simulink subsystem "RoboRio_Controls_sub"  (R2023b)
settings: Solver=VariableStepAuto  StartTime=0.0  StopTime=10.0  RelTol=1e-3
undefined symbols (not defined in the file): All_Num_Poses, All_Paths, Autonomous, Autonomous_lib, Climber_DutyCycle_Neg, Climber_DutyCycle_Pos, FloorDistance, Odometry_IC_X, Odometry_IC_Y
libraries: simulink x5, Disabled_lib x1, Teleop_lib x1, Test_lib x1
(part 1 of 2)
settings Model: Creator=USER  LastModifiedBy=FIRSTMentor

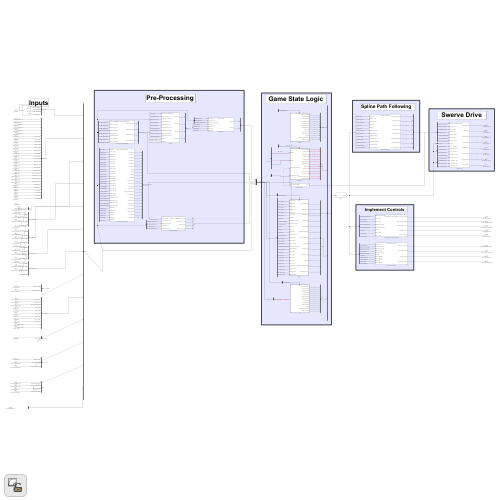
[thumbnail: Simulink's stored preview of the top-level diagram]
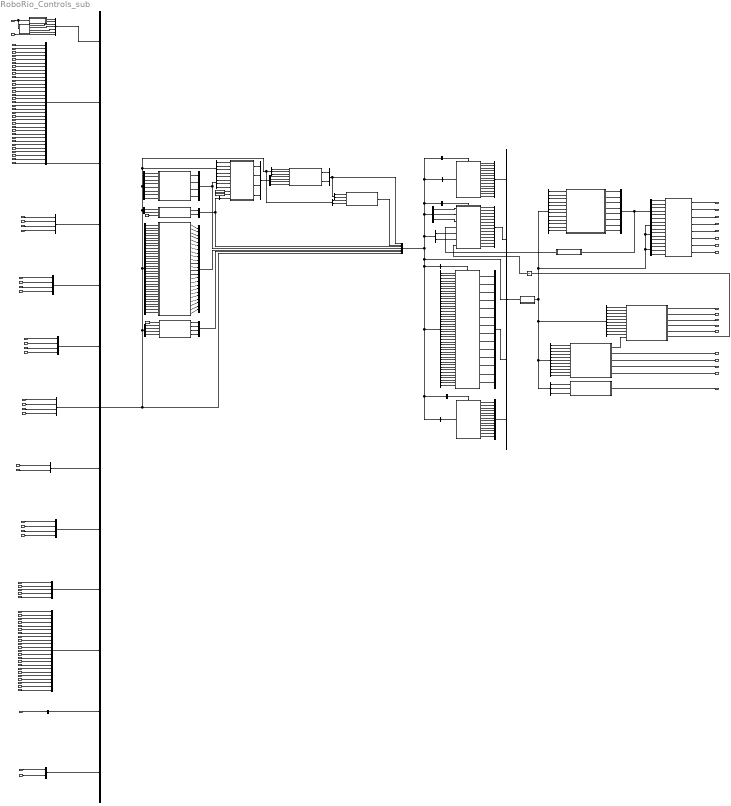
== system RoboRio_Controls_sub ==
  note: Game State Logic
  note: Swerve Drive
  note: Inputs
  note: Pre-Processing
  note: Spline Path
      | Following
  note: Implement Controls
  GameState : Inport
  IsRedAlliance : Inport  Port=2
  Joystick_Left_X : Inport  Port=3
  Joystick_Left_Y : Inport  Port=4
  Joystick_Left_Z : Inport  Port=5
  Joystick_Right_X : Inport  Port=6
  Joystick_Right_Y : Inport  Port=7
  Joystick_Right_Z : Inport  Port=8
  Joystick_Left_B1 : Inport  Port=9
  Joystick_Left_B2 : Inport  Port=10
  Joystick_Left_B3 : Inport  Port=11
  Joystick_Left_B4 : Inport  Port=12
  Joystick_Left_B7 : Inport  Port=13
  Joystick_Left_B8 : Inport  Port=14
  Joystick_Left_B10 : Inport  Port=15
  Joystick_Left_POV : Inport  Port=16
  Joystick_Right_B1 : Inport  Port=17
  Joystick_Right_B2 : Inport  Port=18
  Joystick_Right_B3 : Inport  Port=19
  Joystick_Right_B4 : Inport  Port=20
  Joystick_Right_POV : Inport  Port=21
  Joystick_Right_B7 : Inport  Port=22
  Joystick_Right_B8 : Inport  Port=23
  Joystick_Right_B10 : Inport  Port=24
  Joystick_Right_B14 : Inport  Port=25
  Gamepad_Stick_Left_X : Inport  Port=26
  Gamepad_Stick_Left_Y : Inport  Port=27
  Gamepad_Stick_Right_X : Inport  Port=28
  Gamepad_Stick_Right_Y : Inport  Port=29
  Gamepad_B1_A : Inport  Port=30
  Gamepad_B4_Y : Inport  Port=31
  Gamepad_LB : Inport  Port=32
  Gamepad_LT : Inport  Port=33
  Gamepad_RB : Inport  Port=34
  Gamepad_RT : Inport  Port=35
  Gyro_Angle : Inport  Port=36
  FL_Drive_Motor_Speed : Inport  Port=37
  FR_Drive_Motor_Speed : Inport  Port=38
  BL_Drive_Motor_Speed : Inport  Port=39
  BR_Drive_Motor_Speed : Inport  Port=40
  FL_Drive_Motor_Rev : Inport  Port=41
  FR_Drive_Motor_Rev : Inport  Port=42
  BL_Drive_Motor_Rev : Inport  Port=43
  BR_Drive_Motor_Rev : Inport  Port=44
  FL_Steer_Module_Rev : Inport  Port=45
  FR_Steer_Module_Rev : Inport  Port=46
  BL_Steer_Module_Rev : Inport  Port=47
  BR_Steer_Module_Rev : Inport  Port=48
  FL_Steer_Module_Offset : Inport  Port=49
  FR_Steer_Module_Offset : Inport  Port=50
  BL_Steer_Module_Offset : Inport  Port=51
  BR_Steer_Module_Offset : Inport  Port=52
  Is_Absolute_Steering : Inport  Port=53
  Is_Absolute_Translation : Inport  Port=54
  Intake_TOF_Dist : Inport  Port=55
  Shooter_TOF_Dist : Inport  Port=56
  Shooter_Left_Motor_RPM : Inport  Port=57
  Shooter_Right_Motor_RPM : Inport  Port=58
  Encoder_Revs_Back_Lower : Inport  Port=59
  Encoder_Revs_Back_Upper : Inport  Port=60
  Encoder_Revs_Front : Inport  Port=61
  Encoder_Revs_Ball_Screw : Inport  Port=62
  Encoder_Revs_Climber : Inport  Port=63
  Photon_Est_Pose_X : Inport  Port=64
  Photon_Est_Pose_Y : Inport  Port=65
  Photon_Est_Pose_Ambiguity : Inport  Port=66
  AT_Tag_4_Yaw : Inport  Port=67
  AT_Tag_5_Yaw : Inport  Port=68
  AT_Tag_6_Yaw : Inport  Port=69
  AT_Tag_7_Yaw : Inport  Port=70
  AT_Tag_11_Yaw : Inport  Port=71
  AT_Tag_12_Yaw : Inport  Port=72
  AT_Tag_13_Yaw : Inport  Port=73
  AT_Tag_14_Yaw : Inport  Port=74
  AT_Tag_15_Yaw : Inport  Port=75
  AT_Tag_16_Yaw : Inport  Port=76
  AT_Tag_4_Found : Inport  Port=77
  AT_Tag_5_Found : Inport  Port=78
  AT_Tag_6_Found : Inport  Port=79
  AT_Tag_7_Found : Inport  Port=80
  Line_Sensor_TOF_Range : Inport  Port=81
  AT_Tag_11_Found : Inport  Port=82
  AT_Tag_12_Found : Inport  Port=83
  AT_Tag_13_Found : Inport  Port=84
  AT_Tag_14_Found : Inport  Port=85
  AT_Tag_15_Found : Inport  Port=86
  AT_Tag_16_Found : Inport  Port=87
  Priority_List : Inport  Port=88
  Auto_ID : Inport  Port=89
  Arm_Length_Calculation : Subsystem  ReferencedSubsystem=Arm_Length_Calculation
  Autonomous : Subsystem  AncestorBlock=Autonomous_lib/Autonomous  TreatAsAtomicUnit=on
  Bus Creator : BusCreator  Inputs=7
  Bus Creator{1..2,4,12} (4 alike) : BusCreator  Inputs=14
  Bus Creator{10,19..20,26} (4 alike) : BusCreator  Inputs=2
  Bus Creator11 : BusCreator  Inputs=13
  Bus Creator13 : BusCreator  Inputs=8
  Bus Creator{7..9,14..16,21,23} (8 alike) : BusCreator  Inputs=4
  Bus Creator17 : BusCreator  Inputs=7
  Bus Creator18 : BusCreator  Inputs=23
  Bus Creator22 : BusCreator  Inputs=5
  Bus Creator24 : BusCreator  Inputs=24
  Bus Creator25 : BusCreator  Inputs=1
  Bus Creator3 : BusCreator  Inputs=5
  Bus Creator5 : BusCreator  Inputs=33
  Bus Creator6 : BusCreator  Inputs=1
  Bus Selector : BusSelector  OutputSignals=Steering_Abs_Cmd_SPF,Steering_Rel_Cmd_SPF,Translation_Speed_SPF,Translation_Angle_SPF,Is_Absolute_Translation_SPF,Is_Absolute_Steering_SPF,Gyro_Angle_Adjustment_SPF
  Bus Selector1 : BusSelector  OutputSignals=Odom_Position_X,Odom_Position_Y,Odom_Delta_X,Odom_Delta_Y
  Bus Selector10 : BusSelector  OutputSignals=PreProcessing.Gyro.Gyro_Angle
  Bus Selector11 : BusSelector  OutputSignals=State_Request_Arm,PreProcessing.Arms.Back_Lower_Arm_Length,PreProcessing.Arms.Back_Upper_Arm_Length,PreProcessing.Arms.Front_Arm_Length,PreProcessing.Arms.Ball_Screw_Arm_Length,PreProcessing.Distance_Speaker,Test_Mode,PreProcessing.Human_Inputs.Test_DC_BackUpper,PreProcessing.Human_Inputs.Test_DC_BackLower,PreProcessing.Human_Inputs.Test_DC_Front,PreProcessing.Human_Inputs.Test_DC_BallScrew
  Bus Selector12 : BusSelector  OutputSignals=Human_Inputs.Climber_Cmd_Direction
  Bus Selector13 : BusSelector  OutputSignals=Game_States.GameState,Game_States.Prev_GameState,Human_Inputs.Joystick_Left_X,Human_Inputs.Joystick_Left_Y,Human_Inputs.Joystick_Left_Z,Human_Inputs.Joystick_Right_X,Human_Inputs.Joystick_Right_Y,Human_Inputs.Joystick_Right_Z,Human_Inputs.Joystick_Left_B1,Human_Inputs.Joystick_Left_B2,Human_Inputs.Joystick_Left_B3,Human_Inputs.Joystick_Left_B4,Human_Inputs.Joystick_Left_B7,Human_Inputs.Joystick_Left_B8,Human_Inputs.Joystick_Left_B10,Human_Inputs.Joystick_Left_POV,Human_Inputs.Joystick_Right_B1,Human_Inputs.Joystick_Right_B2,Human_Inputs.Joystick_Right_B3,Human_Inputs.Joystick_Right_B4,Human_Inputs.Joystick_Right_POV,Human_Inputs.Joystick_Right_B7,Human_Inputs.Joystick_Right_B8,Human_Inputs.Joystick_Right_B10,Human_Inputs.Joystick_Right_B14,Human_Inputs.Gamepad_Stick_Left_X,Human_Inputs.Gamepad_Stick_Left_Y,Human_Inputs.Gamepad_Stick_Right_X,Human_Inputs.Gamepad_Stick_Right_Y,Human_Inputs.Gamepad_B1_A,Human_Inputs.Gamepad_B4_Y,Human_Inputs.Gamepad_LB,Human_Inputs.Gamepad_LT,Human_Inputs.Gamepad_RB,Human_Inputs.Gamepad_RT
  Bus Selector14 : BusSelector  OutputSignals=Human_Inputs.State_Request_Arm
  Bus Selector15 : BusSelector  OutputSignals=PreProcessing.Inputs.Game_States.GameState,Climber_Cmd_Direction,PreProcessing.Inputs.Arms.Encoder_Revs_Climber
  Bus Selector16 : BusSelector  OutputSignals=Photon_Estimates.AT_Tag_4_Found,Photon_Estimates.AT_Tag_7_Found
  Bus Selector17 : BusSelector  OutputSignals=IMU_Sensor.Gyro_Angle_deg,Game_States.IsRedAlliance
  Bus Selector18 : BusSelector  OutputSignals=Inputs.Autonomus_Input.Auto_ID,Inputs.Autonomus_Input.Priority_List
  Bus Selector19 : BusSelector  OutputSignals=Gyro_Angle_Field
  Bus Selector2 : BusSelector  OutputSignals=Inputs.Game_States.Game_State_Teleop
  Bus Selector20 : BusSelector  OutputSignals=KF_Position_X,KF_Position_Y
  Bus Selector3 : BusSelector  OutputSignals=Photon_Estimates.Photon_Est_Pose_X,Photon_Estimates.Photon_Est_Pose_Y,Photon_Estimates.Photon_Est_Pose_Ambiguity
  Bus Selector4 : BusSelector  OutputSignals=Inputs.Game_States.Game_State_Auto
  Bus Selector40 : BusSelector  OutputSignals=Drive_Motor_Revs.FL_Drive_Motor_Rev,Drive_Motor_Revs.FR_Drive_Motor_Rev,Drive_Motor_Revs.BL_Drive_Motor_Rev,Drive_Motor_Revs.BR_Drive_Motor_Rev
  Bus Selector41 : BusSelector  OutputSignals=Human_Inputs.Drive_Joystick_X,Human_Inputs.Drive_Joystick_Y,Human_Inputs.Drive_Joystick_Z,Human_Inputs.Drive_Joystick_Z_Mode,Human_Inputs.Steer_Joystick_X,Human_Inputs.Steer_Joystick_Y,Human_Inputs.Steer_Joystick_Z,Human_Inputs.Is_Boosting,Inputs.Motion_Control_Modes.Is_Absolute_Translation,Inputs.Motion_Control_Modes.Is_Absolute_Steering,Human_Inputs.Align_Trap,Human_Inputs.Align_Amp,Human_Inputs.Align_Speaker,Human_Inputs.Face_Toward_Driver,Human_Inputs.Face_Right_Driver,Human_Inputs.Face_Left_Driver,Human_Inputs.Face_Away_Driver,Human_Inputs.State_Request_Intake_Shooter,Human_Inputs.State_Request_Arm,Human_Inputs.Climber_Cmd_Direction,Inputs.Photon_Estimates.AT_Tag_4_Yaw,Inputs.Photon_Estimates.AT_Tag_5_Yaw,Inputs.Photon_Estimates.AT_Tag_6_Yaw,Inputs.Photon_Estimates.AT_Tag_7_Yaw,Inputs.Photon_Estimates.AT_Tag_11_Yaw,Inputs.Photon_Estimates.AT_Tag_12_Yaw,Inputs.Photon_Estimates.AT_Tag_13_Yaw,Inputs.Photon_Estimates.AT_Tag_14_Yaw,Inputs.Photon_Estimates.AT_Tag_15_Yaw,Inputs.Photon_Estimates.AT_Tag_16_Yaw,Inputs.Photon_Estimates.AT_Tag_4_Found,Inputs.Photon_Estimates.AT_Tag_5_Found,Inputs.Photon_Estimates.AT_Tag_6_Found,Inputs.Photon_Estimates.AT_Tag_7_Found,Inputs.Photon_Estimates.AT_Tag_11_Found,Inputs.Photon_Estimates.AT_Tag_12_Found,Inputs.Photon_Estimates.AT_Tag_13_Found,Inputs.Photon_Estimates.AT_Tag_14_Found,Inputs.Photon_Estimates.AT_Tag_15_Found,Inputs.Photon_Estimates.AT_Tag_16_Found,EKF.KF_Position_X,EKF.KF_Position_Y,Inputs.Photon_Estimates.Photon_Est_Pose_Ambiguity,Distance_Speaker,Inputs.Game_States.IsRedAlliance
  Bus Selector5 : BusSelector  OutputSignals=State_Request_Intake_Shooter,PreProcessing.Inputs.Intake_and_Shooter.Intake_TOF_Dist,PreProcessing.Inputs.Intake_and_Shooter.Shooter_TOF_Dist,PreProcessing.Inputs.Intake_and_Shooter.Shooter_Left_Motor_RPM,PreProcessing.Inputs.Intake_and_Shooter.Shooter_Right_Motor_RPM,Test_Mode,PreProcessing.Human_Inputs.Test_DC_Intake,PreProcessing.Human_Inputs.Test_DC_Shooter,PreProcessing.Distance_Speaker,PreProcessing.Arms.Front_Arm_Length
  Bus Selector50 : BusSelector  OutputSignals=PreProcessing.Inputs.Drive_Motor_Speeds.FL_Drive_Motor_Speed,PreProcessing.Inputs.Drive_Motor_Speeds.FR_Drive_Motor_Speed,PreProcessing.Inputs.Drive_Motor_Speeds.BL_Drive_Motor_Speed,PreProcessing.Inputs.Drive_Motor_Speeds.BR_Drive_Motor_Speed
  Bus Selector52 : BusSelector  OutputSignals=PreProcessing.Steer_Module_Angles.FL_Steer_Module_Angle,PreProcessing.Steer_Module_Angles.FR_Steer_Module_Angle,PreProcessing.Steer_Module_Angles.BL_Steer_Module_Angle,PreProcessing.Steer_Module_Angles.BR_Steer_Module_Angle
  Bus Selector57 : BusSelector  OutputSignals=Steer_Module_Revs.FL_Steer_Module_Rev,Steer_Module_Offsets.FL_Steer_Module_Offset,Steer_Module_Revs.FR_Steer_Module_Rev,Steer_Module_Offsets.FR_Steer_Module_Offset,Steer_Module_Revs.BL_Steer_Module_Rev,Steer_Module_Offsets.BL_Steer_Module_Offset,Steer_Module_Revs.BR_Steer_Module_Rev,Steer_Module_Offsets.BR_Steer_Module_Offset
  Bus Selector58 : BusSelector  OutputSignals=FL_Steer_Module_Angle,FR_Steer_Module_Angle,BL_Steer_Module_Angle,BR_Steer_Module_Angle
  Bus Selector59 : BusSelector  OutputSignals=EKF.KF_Position_X,EKF.KF_Position_Y,Inputs.Autonomous.Line_Sensor_TOF_Range
  Bus Selector6 : BusSelector  OutputSignals=Inputs.Game_States.Game_State_Disabled
  Bus Selector7 : BusSelector  OutputSignals=Arms.Encoder_Revs_Back_Lower,Arms.Encoder_Revs_Back_Upper,Arms.Encoder_Revs_Front,Arms.Encoder_Revs_Ball_Screw
  Bus Selector8 : BusSelector  OutputSignals=Inputs.Game_States.Game_State_Test
  Bus Selector9 : BusSelector  OutputSignals=Spline_Enable,Spline_Ref_Poses,Spline_Num_Poses,PreProcessing.EKF.KF_Position_X,PreProcessing.EKF.KF_Position_Y,Steering_Abs_Cmd,Steering_Rel_Cmd,Translation_Speed,Translation_Angle,Is_Absolute_Translation,Is_Absolute_Steering,Gyro_Angle_Adjustment
  Climber_Control : Subsystem
  Constant : Constant  Value=Odometry_IC_X
  Constant1 : Constant  Value=Odometry_IC_Y
  Constant2 : Constant  Value=0
  Constant3 : Constant  Value=0
  Disabled : Disabled_lib/Disabled  SystemSampleTime=-1  VariantActivationTime=update diagram  AllowFlexibleInterface=on  Latency=0  AutoFrameSizeCalculation=off
  Distance_from_Speaker : Subsystem  ReferencedSubsystem=Distance_from_Speaker
  Gyro_Angles : Subsystem  ReferencedSubsystem=Gyro_Angles
  Human_Input_Pre_Processing : Subsystem  ReferencedSubsystem=Human_Input_Pre_Processing
  Intake_Rollers_and_Shooter_Wheels : Subsystem  ReferencedSubsystem=Intake_Rollers_and_Shooter_Wheels
  Internal Feedback : Subsystem
  Kalman_Filter : Subsystem  ReferencedSubsystem=Kalman_Filter_sub
  Merge : Subsystem
  Odometry : Subsystem  ReferencedSubsystem=Odometry_sub
  Previous GameState : Subsystem
  Shooter_Arm_Controls : Subsystem  ReferencedSubsystem=Shooter_Arm_Controls
  Spline_Path_Following : Subsystem  ReferencedSubsystem=Spline_Path_Following_sub
  Steer_Module_Offset_Adjustments : Subsystem  ReferencedSubsystem=Steer_Module_Offset_Adjustments_sub
  Swerve_Drive : Subsystem  ReferencedSubsystem=Swerve_Drive_sub
  Switch Case : SwitchCase  CaseConditions={0,1,2}
  Teleop : Teleop_lib/Teleop  SystemSampleTime=-1  VariantActivationTime=update diagram  AllowFlexibleInterface=on  Latency=0  AutoFrameSizeCalculation=off
  Test : Test_lib/Test  SystemSampleTime=-1  VariantActivationTime=update diagram  AllowFlexibleInterface=on  Latency=0  AutoFrameSizeCalculation=off
  Unit Delay : UnitDelay  SampleTime=-1  HasFrameUpgradeWarning=on
  FL_Drive_Motor_DC : Outport
  FL_Steering_Motor_DC : Outport  Port=2
  FR_Drive_Motor_DC : Outport  Port=3
  BL_Drive_Motor_DC : Outport  Port=4
  FR_Steering_Motor_DC : Outport  Port=5
  BL_Steering_Motor_DC : Outport  Port=6
  BR_Drive_Motor_DC : Outport  Port=7
  BR_Steering_Motor_DC : Outport  Port=8
  Intake_Motor_DutyCycle : Outport  Port=9
  Shooter_Left_Motor_DutyCycle : Outport  Port=10
  Shooter_Right_Motor_DutyCycle : Outport  Port=11
  Shooter_Brake_Enable : Outport  Port=12
  Back_Upper_Arm_DutyCycle : Outport  Port=13
  Shooter_Servo_Position : Outport  Port=14
  Back_Lower_Arm_DutyCycle : Outport  Port=15
  Front_Arm_DutyCycle : Outport  Port=16
  Ball_Screw_Arm_DutyCycle : Outport  Port=17
  Climber_DutyCycle : Outport  Port=18
  wires:
  Teleop/1 -> Bus Creator2/1
  Teleop/2 -> Bus Creator2/2
  Teleop/3 -> Bus Creator2/3
  Teleop/4 -> Bus Creator2/4
  Teleop/5 -> Bus Creator2/5
  Bus Creator4/1 -> Bus Creator3/1  "Disabled"
  Bus Creator1/1 -> Bus Creator3/2  "Autonomous"
  Bus Creator2/1 -> Bus Creator3/4  "Teleop"
  Switch Case/1 -> Bus Creator/3  "Game_State_Disabled"
  Switch Case/2 -> Bus Creator/4  "Game_State_Auto"
  Switch Case/3 -> Bus Creator/5  "Game_State_Teleop"
  GameState/1 -> Previous GameState/1(GameState_in), Switch Case/1  "GameState"
  Bus Creator12/1 -> Bus Creator3/5  "Test"
  Switch Case/4 -> Bus Creator/6  "Game_State_Test"
  Bus Creator5/1 -> Bus Creator11/2  "Human_Inputs"
  Bus Creator6/1 -> Bus Creator11/3  "IMU_Sensor"
  FL_Drive_Motor_Speed/1 -> Bus Creator7/1  "FL_Drive_Motor_Speed"
  FR_Drive_Motor_Speed/1 -> Bus Creator7/2  "FR_Drive_Motor_Speed"
  BL_Drive_Motor_Speed/1 -> Bus Creator7/3  "BL_Drive_Motor_Speed"
  BR_Drive_Motor_Speed/1 -> Bus Creator7/4  "BR_Drive_Motor_Speed"
  FL_Steer_Module_Rev/1 -> Bus Creator8/1  "FL_Steer_Module_Rev"
  BL_Steer_Module_Rev/1 -> Bus Creator8/3  "BL_Steer_Module_Rev"
  BR_Steer_Module_Rev/1 -> Bus Creator8/4  "BR_Steer_Module_Rev"
  FR_Steer_Module_Rev/1 -> Bus Creator8/2  "FR_Steer_Module_Rev"
  Bus Creator7/1 -> Bus Creator11/4  "Drive_Motor_Speeds"
  Bus Creator8/1 -> Bus Creator11/6  "Steer_Module_Revs"
  FL_Steer_Module_Offset/1 -> Bus Creator9/1  "FL_Steer_Module_Offset"
  FR_Steer_Module_Offset/1 -> Bus Creator9/2  "FR_Steer_Module_Offset"
  BL_Steer_Module_Offset/1 -> Bus Creator9/3  "BL_Steer_Module_Offset"
  BR_Steer_Module_Offset/1 -> Bus Creator9/4  "BR_Steer_Module_Offset"
  Bus Creator9/1 -> Bus Creator11/7  "Steer_Module_Offsets"
  Is_Absolute_Steering/1 -> Bus Creator10/1  "Is_Absolute_Steering"
  Is_Absolute_Translation/1 -> Bus Creator10/2  "Is_Absolute_Translation"
  Bus Creator10/1 -> Bus Creator11/8  "Motion_Control_Modes"
  Teleop/6 -> Bus Creator2/6
  Teleop/7 -> Bus Creator2/7
  Autonomous/2(Steering_Abs_Cmd) -> Bus Creator1/2
  Autonomous/4(Translation_Angle) -> Bus Creator1/4
  Autonomous/1(Gyro_Angle_Adjustment) -> Bus Creator1/1
  Autonomous/5(Translation_Speed) -> Bus Creator1/5
  Autonomous/7(Is_Absolute_Steering) -> Bus Creator1/7
  Autonomous/3(Steering_Rel_Cmd) -> Bus Creator1/3
  Autonomous/6(Is_Absolute_Translation) -> Bus Creator1/6
  Disabled/2 -> Bus Creator4/2
  Disabled/4 -> Bus Creator4/4
  Disabled/1 -> Bus Creator4/1
  Disabled/5 -> Bus Creator4/5
  Disabled/7 -> Bus Creator4/7
  Disabled/3 -> Bus Creator4/3
  Disabled/6 -> Bus Creator4/6
  Test/2 -> Bus Creator12/2
  Test/4 -> Bus Creator12/4
  Test/1 -> Bus Creator12/1
  Test/5 -> Bus Creator12/5
  Test/7 -> Bus Creator12/7
  Test/3 -> Bus Creator12/3
  Test/6 -> Bus Creator12/6
  Bus Creator/1 -> Bus Creator11/1  "Game_States"
  Bus Selector2/1 -> Teleop/Action  "<Game_State_Teleop>"
  Bus Selector4/1 -> Autonomous/Action  "<Game_State_Auto>"
  Bus Selector6/1 -> Disabled/Action  "<Game_State_Disabled>"
  Bus Selector8/1 -> Test/Action  "<Game_State_Test>"
  Bus Selector50/4 -> Swerve_Drive/12  "<BR_Drive_Motor_Speed>"
  Bus Selector50/3 -> Swerve_Drive/11  "<BL_Drive_Motor_Speed>"
  Bus Selector50/2 -> Swerve_Drive/10  "<FR_Drive_Motor_Speed>"
  Bus Selector50/1 -> Swerve_Drive/9  "<FL_Drive_Motor_Speed>"
  Swerve_Drive/1 -> FL_Steering_Motor_DC/1
  Swerve_Drive/2 -> FL_Drive_Motor_DC/1
  Swerve_Drive/3 -> FR_Steering_Motor_DC/1
  Swerve_Drive/4 -> FR_Drive_Motor_DC/1
  Swerve_Drive/5 -> BL_Steering_Motor_DC/1
  Swerve_Drive/6 -> BL_Drive_Motor_DC/1
  Swerve_Drive/7 -> BR_Steering_Motor_DC/1
  Swerve_Drive/8 -> BR_Drive_Motor_DC/1
  Joystick_Left_B1/1 -> Bus Creator5/7  "Joystick_Left_B1"
  Bus Creator14/1 -> Bus Creator11/5  "Drive_Motor_Revs"
  FL_Drive_Motor_Rev/1 -> Bus Creator14/1  "FL_Drive_Motor_Rev"
  FR_Drive_Motor_Rev/1 -> Bus Creator14/2  "FR_Drive_Motor_Rev"
  BL_Drive_Motor_Rev/1 -> Bus Creator14/3  "BL_Drive_Motor_Rev"
  BR_Drive_Motor_Rev/1 -> Bus Creator14/4  "BR_Drive_Motor_Rev"
  Bus Selector40/1 -> Odometry/1  "<FL_Drive_Motor_Rev>"
  Bus Selector40/2 -> Odometry/2  "<FR_Drive_Motor_Rev>"
  Bus Selector40/3 -> Odometry/3  "<BL_Drive_Motor_Rev>"
  Bus Selector40/4 -> Odometry/4  "<BR_Drive_Motor_Rev>"
  Constant1/1 -> Odometry/10
  Constant/1 -> Odometry/9
  Bus Selector57/1 -> Steer_Module_Offset_Adjustments/1  "<FL_Steer_Module_Rev>"
  Bus Selector57/2 -> Steer_Module_Offset_Adjustments/2  "<FL_Steer_Module_Offset>"
  Bus Selector57/3 -> Steer_Module_Offset_Adjustments/3  "<FR_Steer_Module_Rev>"
  Bus Selector57/4 -> Steer_Module_Offset_Adjustments/4  "<FR_Steer_Module_Offset>"
  Bus Selector57/5 -> Steer_Module_Offset_Adjustments/5  "<BL_Steer_Module_Rev>"
  Bus Selector57/6 -> Steer_Module_Offset_Adjustments/6  "<BL_Steer_Module_Offset>"
  Bus Selector57/7 -> Steer_Module_Offset_Adjustments/7  "<BR_Steer_Module_Rev>"
  Bus Selector57/8 -> Steer_Module_Offset_Adjustments/8  "<BR_Steer_Module_Offset>"
  Steer_Module_Offset_Adjustments/2 -> Bus Creator15/2
  Steer_Module_Offset_Adjustments/1 -> Bus Creator15/1
  Steer_Module_Offset_Adjustments/3 -> Bus Creator15/3
  Steer_Module_Offset_Adjustments/4 -> Bus Creator15/4
  Bus Creator15/1 -> Bus Selector58/1, Bus Creator17/4  "Steer_Module_Angles"
  Bus Selector58/1 -> Odometry/5  "<FL_Steer_Module_Angle>"
  Bus Selector58/2 -> Odometry/6  "<FR_Steer_Module_Angle>"
  Bus Selector58/3 -> Odometry/7  "<BL_Steer_Module_Angle>"
  Bus Selector58/4 -> Odometry/8  "<BR_Steer_Module_Angle>"
  Bus Creator16/1 -> Bus Selector1/1  "Odometry"
  Bus Creator11/1 -> Bus Creator17/7, Bus Selector7/1, Bus Selector13/1, Bus Selector57/1, Bus Selector40/1, Bus Selector3/1, Bus Selector16/1, Bus Selector17/1  "Inputs"
  Bus Selector52/1 -> Swerve_Drive/13  "<FL_Steer_Module_Angle>"
  Bus Selector52/2 -> Swerve_Drive/14  "<FR_Steer_Module_Angle>"
  Bus Selector52/3 -> Swerve_Drive/15  "<BL_Steer_Module_Angle>"
  Bus Selector52/4 -> Swerve_Drive/16  "<BR_Steer_Module_Angle>"
  Disabled/8 -> Bus Creator4/8
  Disabled/9 -> Bus Creator4/9
  Disabled/10 -> Bus Creator4/10
  Autonomous/8(Spline_Enable) -> Bus Creator1/8
  Autonomous/9(Spline_Ref_Poses) -> Bus Creator1/9
  Autonomous/10(Spline_Num_Poses) -> Bus Creator1/10
  Teleop/8 -> Bus Creator2/8
  Teleop/9 -> Bus Creator2/9
  Teleop/10 -> Bus Creator2/10
  Test/8 -> Bus Creator12/8
  Test/9 -> Bus Creator12/9
  Test/10 -> Bus Creator12/10
  Merge/1(Bus_Out) -> Bus Selector5/1, Bus Selector11/1, Bus Selector15/1, Bus Selector52/1, Bus Selector50/1, Bus Selector10/1, Bus Selector9/1
  Bus Creator3/1 -> Merge/1(Bus_In)
  Bus Selector10/1 -> Swerve_Drive/8  "<Gyro_Angle>"
  Bus Selector59/1 -> Autonomous/1(Chassis_X)  "<KF_Position_X>"
  Bus Selector59/2 -> Autonomous/2(Chassis_Y)  "<KF_Position_Y>"
  Bus Selector9/1 -> Spline_Path_Following/1  "<Spline_Enable>"
  Bus Selector9/2 -> Spline_Path_Following/2  "<Spline_Ref_Poses>"
  Bus Selector9/3 -> Spline_Path_Following/3  "<Spline_Num_Poses>"
  Bus Selector9/6 -> Spline_Path_Following/6  "<Steering_Abs_Cmd>"
  Bus Selector9/7 -> Spline_Path_Following/7  "<Steering_Rel_Cmd>"
  Bus Selector9/8 -> Spline_Path_Following/8  "<Translation_Speed>"
  Bus Selector9/9 -> Spline_Path_Following/9  "<Translation_Angle>"
  Bus Selector9/10 -> Spline_Path_Following/10  "<Is_Absolute_Translation>"
  Bus Selector9/11 -> Spline_Path_Following/11  "<Is_Absolute_Steering>"
  Bus Selector9/12 -> Spline_Path_Following/12  "<Gyro_Angle_Adjustment>"
  Spline_Path_Following/2 -> Bus Creator13/2
  Spline_Path_Following/3 -> Bus Creator13/3
  Spline_Path_Following/4 -> Bus Creator13/4
  Spline_Path_Following/5 -> Bus Creator13/5
  Spline_Path_Following/6 -> Bus Creator13/6
  Spline_Path_Following/7 -> Bus Creator13/7
  Spline_Path_Following/8 -> Bus Creator13/8
  Bus Creator13/1 -> Internal Feedback/1(Bus_In), Bus Selector/1
  Bus Selector/5 -> Swerve_Drive/5  "<Is_Absolute_Translation_SPF>"
  Bus Selector/4 -> Swerve_Drive/4  "<Translation_Angle_SPF>"
  Bus Selector/6 -> Swerve_Drive/6  "<Is_Absolute_Steering_SPF>"
  Bus Selector/3 -> Swerve_Drive/3  "<Translation_Speed_SPF>"
  Bus Selector/7 -> Swerve_Drive/7  "<Gyro_Angle_Adjustment_SPF>"
  Bus Selector/2 -> Swerve_Drive/2  "<Steering_Rel_Cmd_SPF>"
  Bus Selector/1 -> Swerve_Drive/1  "<Steering_Abs_Cmd_SPF>"
  Spline_Path_Following/1 -> Bus Creator13/1
  Photon_Est_Pose_X/1 -> Bus Creator18/1  "Photon_Est_Pose_X"
  Photon_Est_Pose_Y/1 -> Bus Creator18/2  "Photon_Est_Pose_Y"
  Photon_Est_Pose_Ambiguity/1 -> Bus Creator18/3  "Photon_Est_Pose_Ambiguity"
  Bus Selector1/3 -> Kalman_Filter/6  "<Odom_Delta_X>"
  Bus Selector1/4 -> Kalman_Filter/7  "<Odom_Delta_Y>"
  Bus Selector3/3 -> Kalman_Filter/3  "<Photon_Est_Pose_Ambiguity>"
  Bus Selector3/2 -> Kalman_Filter/2  "<Photon_Est_Pose_Y>"
  Bus Selector3/1 -> Kalman_Filter/1  "<Photon_Est_Pose_X>"
  Kalman_Filter/1 -> Bus Creator19/1
  Kalman_Filter/2 -> Bus Creator19/2
  Bus Selector9/4 -> Spline_Path_Following/4  "<KF_Position_X>"
  Bus Selector9/5 -> Spline_Path_Following/5  "<KF_Position_Y>"
  Bus Creator19/1 -> Bus Selector20/1, Bus Creator17/1  "EKF"
  Odometry/1 -> Bus Creator16/1
  Odometry/2 -> Bus Creator16/2
  Odometry/3 -> Bus Creator16/3
  Odometry/4 -> Bus Creator16/4
  Bus Selector1/2 -> Kalman_Filter/5  "<Odom_Position_Y>"
  Bus Selector1/1 -> Kalman_Filter/4  "<Odom_Position_X>"
  Bus Selector5/2 -> Intake_Rollers_and_Shooter_Wheels/2  "<Intake_TOF_Dist>"
  Intake_Rollers_and_Shooter_Wheels/1 -> Intake_Motor_DutyCycle/1
  Shooter_TOF_Dist/1 -> Bus Creator21/2  "Shooter_TOF_Dist"
  Shooter_Left_Motor_RPM/1 -> Bus Creator21/3  "Shooter_Left_Motor_RPM"
  Shooter_Right_Motor_RPM/1 -> Bus Creator21/4  "Shooter_Right_Motor_RPM"
  Bus Selector5/3 -> Intake_Rollers_and_Shooter_Wheels/3  "<Shooter_TOF_Dist>"
  Bus Selector5/4 -> Intake_Rollers_and_Shooter_Wheels/4  "<Shooter_Left_Motor_RPM>"
  Bus Selector5/5 -> Intake_Rollers_and_Shooter_Wheels/5  "<Shooter_Right_Motor_RPM>"
  Intake_Rollers_and_Shooter_Wheels/2 -> Shooter_Left_Motor_DutyCycle/1
  Intake_Rollers_and_Shooter_Wheels/3 -> Shooter_Right_Motor_DutyCycle/1
  Intake_Rollers_and_Shooter_Wheels/4 -> Shooter_Brake_Enable/1
  Intake_Rollers_and_Shooter_Wheels/5 -> Shooter_Servo_Position/1
  Encoder_Revs_Back_Lower/1 -> Bus Creator22/1  "Encoder_Revs_Back_Lower"
  Encoder_Revs_Back_Upper/1 -> Bus Creator22/2  "Encoder_Revs_Back_Upper"
  Encoder_Revs_Front/1 -> Bus Creator22/3  "Encoder_Revs_Front"
  Encoder_Revs_Ball_Screw/1 -> Bus Creator22/4  "Encoder_Revs_Ball_Screw"
  Arm_Length_Calculation/1 -> Bus Creator23/1
  Arm_Length_Calculation/2 -> Bus Creator23/2
  Arm_Length_Calculation/3 -> Bus Creator23/3
  Arm_Length_Calculation/4 -> Bus Creator23/4
  Bus Creator23/1 -> Bus Creator17/6  "Arms"
  Bus Selector11/2 -> Shooter_Arm_Controls/2  "<Back_Lower_Arm_Length>"
  Bus Selector11/3 -> Shooter_Arm_Controls/3  "<Back_Upper_Arm_Length>"
  Bus Selector11/4 -> Shooter_Arm_Controls/4  "<Front_Arm_Length>"
  Bus Selector11/5 -> Shooter_Arm_Controls/5  "<Ball_Screw_Arm_Length>"
  Shooter_Arm_Controls/2 -> Back_Upper_Arm_DutyCycle/1
  Shooter_Arm_Controls/3 -> Back_Lower_Arm_DutyCycle/1
  Shooter_Arm_Controls/4 -> Front_Arm_DutyCycle/1
  Shooter_Arm_Controls/5 -> Ball_Screw_Arm_DutyCycle/1
  Bus Selector7/1 -> Arm_Length_Calculation/2  "<Encoder_Revs_Back_Lower>"
  Bus Selector7/2 -> Arm_Length_Calculation/3  "<Encoder_Revs_Back_Upper>"
  Bus Selector7/3 -> Arm_Length_Calculation/4  "<Encoder_Revs_Front>"
  Bus Selector7/4 -> Arm_Length_Calculation/5  "<Encoder_Revs_Ball_Screw>"
  Test/11 -> Bus Creator12/11
  Teleop/11 -> Bus Creator2/11
  Autonomous/11(Test_Mode) -> Bus Creator1/11
  Disabled/11 -> Bus Creator4/11
  Joystick_Right_B4/1 -> Bus Creator5/18  "Joystick_Right_B4"
  Joystick_Right_B3/1 -> Bus Creator5/17  "Joystick_Right_B3"
  Joystick_Right_B2/1 -> Bus Creator5/16  "Joystick_Right_B2"
  Joystick_Right_B1/1 -> Bus Creator5/15  "Joystick_Right_B1"
  Joystick_Left_B10/1 -> Bus Creator5/13  "Joystick_Left_B10"
  Joystick_Left_B8/1 -> Bus Creator5/12  "Joystick_Left_B8"
  Joystick_Left_B4/1 -> Bus Creator5/10  "Joystick_Left_B4"
  Joystick_Left_B3/1 -> Bus Creator5/9  "Joystick_Left_B3"
  Joystick_Left_B2/1 -> Bus Creator5/8  "Joystick_Left_B2"
  Bus Selector13/6 -> Human_Input_Pre_Processing/6  "<Joystick_Right_X>"
  Bus Selector13/7 -> Human_Input_Pre_Processing/7  "<Joystick_Right_Y>"
  Bus Selector13/3 -> Human_Input_Pre_Processing/3  "<Joystick_Left_X>"
  Bus Selector13/5 -> Human_Input_Pre_Processing/5  "<Joystick_Left_Z>"
  Bus Selector13/4 -> Human_Input_Pre_Processing/4  "<Joystick_Left_Y>"
  Bus Selector13/8 -> Human_Input_Pre_Processing/8  "<Joystick_Right_Z>"
  Bus Selector13/9 -> Human_Input_Pre_Processing/9  "<Joystick_Left_B1>"
  Bus Selector13/10 -> Human_Input_Pre_Processing/10  "<Joystick_Left_B2>"
  Bus Selector13/11 -> Human_Input_Pre_Processing/11  "<Joystick_Left_B3>"
  Bus Selector13/12 -> Human_Input_Pre_Processing/12  "<Joystick_Left_B4>"
  Bus Selector13/14 -> Human_Input_Pre_Processing/14  "<Joystick_Left_B8>"
  Bus Selector13/15 -> Human_Input_Pre_Processing/15  "<Joystick_Left_B10>"
  Bus Selector13/17 -> Human_Input_Pre_Processing/17  "<Joystick_Right_B1>"
  Bus Selector13/18 -> Human_Input_Pre_Processing/18  "<Joystick_Right_B2>"
  Bus Selector13/19 -> Human_Input_Pre_Processing/19  "<Joystick_Right_B3>"
  Bus Selector13/20 -> Human_Input_Pre_Processing/20  "<Joystick_Right_B4>"
  Bus Selector13/23 -> Human_Input_Pre_Processing/23  "<Joystick_Right_B8>"
  Bus Selector13/24 -> Human_Input_Pre_Processing/24  "<Joystick_Right_B10>"
  Bus Selector13/27 -> Human_Input_Pre_Processing/27  "<Gamepad_Stick_Left_Y>"
  Bus Selector13/29 -> Human_Input_Pre_Processing/29  "<Gamepad_Stick_Right_Y>"
  Bus Selector13/30 -> Human_Input_Pre_Processing/30  "<Gamepad_B1_A>"
  Bus Selector13/32 -> Human_Input_Pre_Processing/32  "<Gamepad_LB>"
  Bus Selector13/33 -> Human_Input_Pre_Processing/33  "<Gamepad_LT>"
  Bus Selector13/34 -> Human_Input_Pre_Processing/34  "<Gamepad_RB>"
  Bus Selector13/35 -> Human_Input_Pre_Processing/35  "<Gamepad_RT>"
  Joystick_Left_Y/1 -> Bus Creator5/2  "Joystick_Left_Y"
  Joystick_Left_X/1 -> Bus Creator5/1  "Joystick_Left_X"
  Joystick_Left_Z/1 -> Bus Creator5/3  "Joystick_Left_Z"
  Joystick_Right_X/1 -> Bus Creator5/4  "Joystick_Right_X"
  Joystick_Right_Y/1 -> Bus Creator5/5  "Joystick_Right_Y"
  Joystick_Right_Z/1 -> Bus Creator5/6  "Joystick_Right_Z"
  Gamepad_Stick_Left_Y/1 -> Bus Creator5/25  "Gamepad_Stick_Left_Y"
  Joystick_Right_B10/1 -> Bus Creator5/22  "Joystick_Right_B10"
  Gamepad_Stick_Right_Y/1 -> Bus Creator5/27  "Gamepad_Stick_Right_Y"
  Joystick_Right_B8/1 -> Bus Creator5/21  "Joystick_Right_B8"
  Gamepad_B1_A/1 -> Bus Creator5/28  "Gamepad_B1_A"
  Joystick_Right_POV/1 -> Bus Creator5/19  "Joystick_Right_POV"
  Gamepad_LB/1 -> Bus Creator5/30  "Gamepad_LB"
  Gamepad_LT/1 -> Bus Creator5/31  "Gamepad_LT"
  Gamepad_RB/1 -> Bus Creator5/32  "Gamepad_RB"
  Gamepad_RT/1 -> Bus Creator5/33  "Gamepad_RT"
  Bus Selector13/21 -> Human_Input_Pre_Processing/21  "<Joystick_Right_POV>"
  Human_Input_Pre_Processing/1 -> Bus Creator24/1
  Human_Input_Pre_Processing/2 -> Bus Creator24/2
  Human_Input_Pre_Processing/3 -> Bus Creator24/3
  Human_Input_Pre_Processing/5 -> Bus Creator24/5
  Human_Input_Pre_Processing/6 -> Bus Creator24/6
  Human_Input_Pre_Processing/7 -> Bus Creator24/7
  Human_Input_Pre_Processing/8 -> Bus Creator24/8
  Human_Input_Pre_Processing/9 -> Bus Creator24/9
  Human_Input_Pre_Processing/10 -> Bus Creator24/10
  Human_Input_Pre_Processing/11 -> Bus Creator24/11
  Human_Input_Pre_Processing/12 -> Bus Creator24/12
  Human_Input_Pre_Processing/13 -> Bus Creator24/13
  Human_Input_Pre_Processing/14 -> Bus Creator24/14
  Human_Input_Pre_Processing/15 -> Bus Creator24/15
  Human_Input_Pre_Processing/16 -> Bus Creator24/16
  Human_Input_Pre_Processing/17 -> Bus Creator24/17
  Bus Creator24/1 -> Bus Creator17/5  "Human_Inputs"
  Bus Selector41/1 -> Teleop/1  "<Drive_Joystick_X>"
  Bus Selector41/2 -> Teleop/2  "<Drive_Joystick_Y>"
  Bus Selector41/3 -> Teleop/3  "<Drive_Joystick_Z>"
  Gamepad_B4_Y/1 -> Bus Creator5/29  "Gamepad_B4_Y"
  Bus Selector13/31 -> Human_Input_Pre_Processing/31  "<Gamepad_B4_Y>"
  Disabled/12 -> Bus Creator4/12
  Disabled/13 -> Bus Creator4/13
  Autonomous/12(State_Request_Intake_Shooter) -> Bus Creator1/12
  Autonomous/13(State_Request_Arm) -> Bus Creator1/13
  Teleop/12 -> Bus Creator2/12
  Teleop/13 -> Bus Creator2/13
  Test/12 -> Bus Creator12/12
  Test/13 -> Bus Creator12/13
  Bus Selector11/1 -> Shooter_Arm_Controls/1  "<State_Request_Arm>"
  Bus Selector5/1 -> Intake_Rollers_and_Shooter_Wheels/1  "<State_Request_Intake_Shooter>"
  AT_Tag_4_Yaw/1 -> Bus Creator18/4  "AT_Tag_4_Yaw"
  AT_Tag_5_Yaw/1 -> Bus Creator18/5  "AT_Tag_5_Yaw"
  AT_Tag_6_Yaw/1 -> Bus Creator18/6  "AT_Tag_6_Yaw"
  AT_Tag_7_Yaw/1 -> Bus Creator18/7  "AT_Tag_7_Yaw"
  Bus Selector13/1 -> Human_Input_Pre_Processing/1  "<GameState>"
  Bus Selector11/7 -> Shooter_Arm_Controls/7  "<Test_Mode>"
  Bus Selector11/9 -> Shooter_Arm_Controls/9  "<Test_DC_BackLower>"
  Bus Selector11/8 -> Shooter_Arm_Controls/8  "<Test_DC_BackUpper>"
  Bus Selector11/10 -> Shooter_Arm_Controls/10  "<Test_DC_Front>"
  Bus Selector11/11 -> Shooter_Arm_Controls/11  "<Test_DC_BallScrew>"
  Bus Selector5/6 -> Intake_Rollers_and_Shooter_Wheels/6  "<Test_Mode>"
  Bus Selector5/7 -> Intake_Rollers_and_Shooter_Wheels/7  "<Test_DC_Intake>"
  Bus Selector5/8 -> Intake_Rollers_and_Shooter_Wheels/8  "<Test_DC_Shooter>"
  Gamepad_Stick_Left_X/1 -> Bus Creator5/24  "Gamepad_Stick_Left_X"
  Gamepad_Stick_Right_X/1 -> Bus Creator5/26  "Gamepad_Stick_Right_X"
  Bus Selector13/26 -> Human_Input_Pre_Processing/26  "<Gamepad_Stick_Left_X>"
  Bus Selector13/28 -> Human_Input_Pre_Processing/28  "<Gamepad_Stick_Right_X>"
  Bus Creator17/1 -> Bus Selector18/1, Bus Selector59/1, Bus Selector4/1, Bus Selector14/1, Bus Selector6/1, Bus Creator3/3, Bus Selector2/1, Bus Selector41/1, Bus Selector8/1, Bus Selector12/1  "PreProcessing"
  Intake_TOF_Dist/1 -> Bus Creator21/1  "Intake_TOF_Dist"
  Line_Sensor_TOF_Range/1 -> Bus Creator25/1  "Line_Sensor_TOF_Range"
  Bus Creator21/1 -> Bus Creator11/9  "Intake_and_Shooter"
  Bus Creator22/1 -> Bus Creator11/10  "Arms"
  Bus Creator18/1 -> Bus Creator11/11  "Photon_Estimates"
  Bus Creator25/1 -> Bus Creator11/12  "Autonomous"
  Internal Feedback/1(Robot_Reached_Destination) -> Autonomous/4(Robot_Reached_Destination)
  Bus Selector59/3 -> Autonomous/3(Line_Sensor_TOF_Range)  "<Line_Sensor_TOF_Range>"
  AT_Tag_11_Yaw/1 -> Bus Creator18/8  "AT_Tag_11_Yaw"
  AT_Tag_12_Yaw/1 -> Bus Creator18/9  "AT_Tag_12_Yaw"
  AT_Tag_13_Yaw/1 -> Bus Creator18/10  "AT_Tag_13_Yaw"
  AT_Tag_14_Yaw/1 -> Bus Creator18/11  "AT_Tag_14_Yaw"
  AT_Tag_15_Yaw/1 -> Bus Creator18/12  "AT_Tag_15_Yaw"
  AT_Tag_16_Yaw/1 -> Bus Creator18/13  "AT_Tag_16_Yaw"
  AT_Tag_4_Found/1 -> Bus Creator18/14  "AT_Tag_4_Found"
  AT_Tag_5_Found/1 -> Bus Creator18/15  "AT_Tag_5_Found"
  AT_Tag_6_Found/1 -> Bus Creator18/16  "AT_Tag_6_Found"
  AT_Tag_7_Found/1 -> Bus Creator18/17  "AT_Tag_7_Found"
  AT_Tag_11_Found/1 -> Bus Creator18/18  "AT_Tag_11_Found"
  AT_Tag_12_Found/1 -> Bus Creator18/19  "AT_Tag_12_Found"
  AT_Tag_13_Found/1 -> Bus Creator18/20  "AT_Tag_13_Found"
  AT_Tag_14_Found/1 -> Bus Creator18/21  "AT_Tag_14_Found"
  AT_Tag_15_Found/1 -> Bus Creator18/22  "AT_Tag_15_Found"
  AT_Tag_16_Found/1 -> Bus Creator18/23  "AT_Tag_16_Found"
  Joystick_Left_B7/1 -> Bus Creator5/11  "Joystick_Left_B7"
  Joystick_Right_B7/1 -> Bus Creator5/20  "Joystick_Right_B7"
  Bus Selector13/22 -> Human_Input_Pre_Processing/22  "<Joystick_Right_B7>"
  Bus Selector13/13 -> Human_Input_Pre_Processing/13  "<Joystick_Left_B7>"
  Human_Input_Pre_Processing/18 -> Bus Creator24/18
  Teleop/14 -> Bus Creator2/14
  Test/14 -> Bus Creator12/14
  Bus Selector12/1 -> Test/1  "<Climber_Cmd_Direction>"
  Disabled/14 -> Bus Creator4/14
  Autonomous/14(Climber_Cmd_Direction) -> Bus Creator1/14
  Previous GameState/1(GameState) -> Bus Creator/1
  Previous GameState/2(Prev_GameState) -> Bus Creator/2
  Bus Selector13/2 -> Human_Input_Pre_Processing/2  "<Prev_GameState>"
  Bus Selector16/1 -> Distance_from_Speaker/3  "<AT_Tag_4_Found>"
  Bus Selector16/2 -> Distance_from_Speaker/4  "<AT_Tag_7_Found>"
  Gyro_Angle/1 -> Bus Creator6/1  "Gyro_Angle_deg"
  IsRedAlliance/1 -> Bus Creator/7  "IsRedAlliance"
  Bus Selector17/2 -> Gyro_Angles/2  "<IsRedAlliance>"
  Bus Selector17/1 -> Gyro_Angles/1  "<Gyro_Angle_deg>"
  Gyro_Angles/1 -> Bus Creator20/1
  Gyro_Angles/2 -> Bus Creator20/2
  Bus Creator20/1 -> Bus Selector19/1, Bus Creator17/3  "Gyro"
  Bus Selector19/1 -> Odometry/11  "<Gyro_Angle_Field>"
  Bus Selector20/1 -> Distance_from_Speaker/1  "<KF_Position_X>"
  Bus Selector20/2 -> Distance_from_Speaker/2  "<KF_Position_Y>"
  Distance_from_Speaker/1 -> Bus Creator17/2
  Constant2/1 -> Arm_Length_Calculation/1  "Arm_Dist_Cal_Flag"
  Joystick_Right_B14/1 -> Bus Creator5/23  "Joystick_Right_B14"
  Bus Selector13/25 -> Human_Input_Pre_Processing/25  "<Joystick_Right_B14>"
  Bus Selector14/1 -> Disabled/1  "<State_Request_Arm>"
  Constant3/1 -> Gyro_Angles/3
  Joystick_Left_POV/1 -> Bus Creator5/14  "Joystick_Left_POV"
  Bus Selector13/16 -> Human_Input_Pre_Processing/16  "<Joystick_Left_POV>"
  Human_Input_Pre_Processing/19 -> Bus Creator24/19
  Human_Input_Pre_Processing/20 -> Bus Creator24/20
  Human_Input_Pre_Processing/21 -> Bus Creator24/21
  Human_Input_Pre_Processing/22 -> Bus Creator24/22
  Human_Input_Pre_Processing/23 -> Bus Creator24/23
  Human_Input_Pre_Processing/24 -> Bus Creator24/24
  Human_Input_Pre_Processing/4 -> Bus Creator24/4
  Bus Selector41/4 -> Teleop/4  "<Drive_Joystick_Z_Mode>"
  Bus Selector41/5 -> Teleop/5  "<Steer_Joystick_X>"
  Bus Selector41/6 -> Teleop/6  "<Steer_Joystick_Y>"
  Bus Selector41/7 -> Teleop/7  "<Steer_Joystick_Z>"
  Bus Selector41/8 -> Teleop/8  "<Is_Boosting>"
  Bus Selector41/9 -> Teleop/9  "<Is_Absolute_Translation>"
  Bus Selector41/10 -> Teleop/10  "<Is_Absolute_Steering>"
  Bus Selector41/11 -> Teleop/11  "<Align_Trap>"
  Bus Selector41/12 -> Teleop/12  "<Align_Amp>"
  Bus Selector41/13 -> Teleop/13  "<Align_Speaker>"
  Bus Selector41/14 -> Teleop/14  "<Face_Toward_Driver>"
  Bus Selector41/15 -> Teleop/15  "<Face_Right_Driver>"
  Bus Selector41/16 -> Teleop/16  "<Face_Left_Driver>"
  Bus Selector41/17 -> Teleop/17  "<Face_Away_Driver>"
  Bus Selector41/18 -> Teleop/18  "<State_Request_Intake_Shooter>"
  Bus Selector41/19 -> Teleop/19  "<State_Request_Arm>"
  Bus Selector41/20 -> Teleop/20  "<Climber_Cmd_Direction>"
  Bus Selector41/21 -> Teleop/21  "<AT_Tag_4_Yaw>"
  Bus Selector41/22 -> Teleop/22  "<AT_Tag_5_Yaw>"
  Bus Selector41/23 -> Teleop/23  "<AT_Tag_6_Yaw>"
  Bus Selector41/24 -> Teleop/24  "<AT_Tag_7_Yaw>"
  Bus Selector41/25 -> Teleop/25  "<AT_Tag_11_Yaw>"
  Bus Selector41/26 -> Teleop/26  "<AT_Tag_12_Yaw>"
  Bus Selector41/27 -> Teleop/27  "<AT_Tag_13_Yaw>"
  Bus Selector41/28 -> Teleop/28  "<AT_Tag_14_Yaw>"
  Bus Selector41/29 -> Teleop/29  "<AT_Tag_15_Yaw>"
  Bus Selector41/30 -> Teleop/30  "<AT_Tag_16_Yaw>"
  Bus Selector41/31 -> Teleop/31  "<AT_Tag_4_Found>"
  Bus Selector41/32 -> Teleop/32  "<AT_Tag_5_Found>"
  Bus Selector41/33 -> Teleop/33  "<AT_Tag_6_Found>"
  Bus Selector41/34 -> Teleop/34  "<AT_Tag_7_Found>"
  Bus Selector41/35 -> Teleop/35  "<AT_Tag_11_Found>"
  Bus Selector41/36 -> Teleop/36  "<AT_Tag_12_Found>"
  Bus Selector41/37 -> Teleop/37  "<AT_Tag_13_Found>"
  Bus Selector41/38 -> Teleop/38  "<AT_Tag_14_Found>"
  Bus Selector41/39 -> Teleop/39  "<AT_Tag_15_Found>"
  Bus Selector41/40 -> Teleop/40  "<AT_Tag_16_Found>"
  Bus Selector41/41 -> Teleop/41  "<KF_Position_X>"
  Bus Selector41/42 -> Teleop/42  "<KF_Position_Y>"
  Bus Selector41/43 -> Teleop/43  "<Photon_Est_Pose_Ambiguity>"
  Bus Selector41/44 -> Teleop/44  "<Distance_Speaker>"
  Bus Selector41/45 -> Teleop/45  "<IsRedAlliance>"
  Bus Selector11/6 -> Shooter_Arm_Controls/6  "<Distance_Speaker>"
  Shooter_Arm_Controls/1 -> Intake_Rollers_and_Shooter_Wheels/11
  Bus Selector5/9 -> Intake_Rollers_and_Shooter_Wheels/9  "<Distance_Speaker>"
  Intake_Rollers_and_Shooter_Wheels/6 -> Unit Delay/1
  Unit Delay/1 -> Autonomous/7(IsWaitingForCommand)
  Priority_List/1 -> Bus Creator26/1  "Priority_List"
  Auto_ID/1 -> Bus Creator26/2  "Auto_ID"
  Bus Creator26/1 -> Bus Creator11/13  "Autonomus_Input"
  Bus Selector18/1 -> Autonomous/5(Auto_ID)  "<Auto_ID>"
  Bus Selector18/2 -> Autonomous/6(PriorityList)  "<Priority_List>"
  Bus Selector5/10 -> Intake_Rollers_and_Shooter_Wheels/10  "<Front_Arm_Length>"
  Bus Selector15/2 -> Climber_Control/2(Climber_Cmd_Direction)  "<Climber_Cmd_Direction>"
  Bus Selector15/3 -> Climber_Control/3(Encoder_Revs_Climber)  "<Encoder_Revs_Climber>"
  Climber_Control/1(Climber_DutyCyce) -> Climber_DutyCycle/1
  Encoder_Revs_Climber/1 -> Bus Creator22/5  "Encoder_Revs_Climber"
  Bus Selector15/1 -> Climber_Control/1(GameState)  "<GameState>"

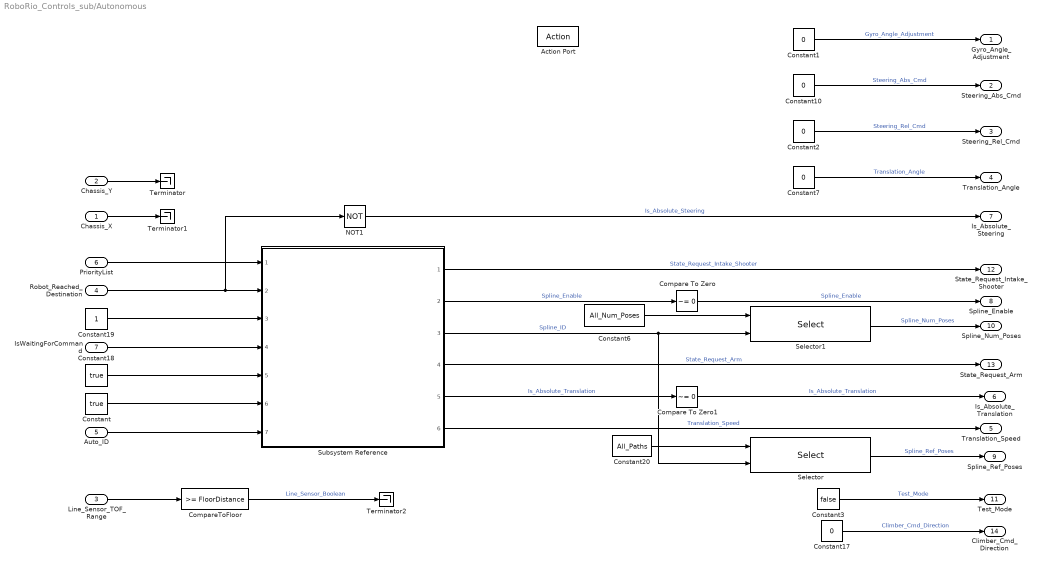
== system RoboRio_Controls_sub/Autonomous ==
  Chassis_X : Inport
  Chassis_Y : Inport  Port=2
  Line_Sensor_TOF_Range : Inport  Port=3
  Robot_Reached_Destination : Inport  Port=4
  Auto_ID : Inport  Port=5
  PriorityList : Inport  Port=6
  IsWaitingForCommand : Inport  Port=7
  Action Port : ActionPort  InitializeStates=reset
  Compare To Zero : simulink/Logic and Bit Operations/Compare To Zero  relop=~=  OutDataTypeStr=boolean
  Compare To Zero1 : simulink/Logic and Bit Operations/Compare To Zero  relop=~=  OutDataTypeStr=boolean
  CompareToFloor : simulink/Logic and Bit Operations/Compare To Constant  relop=>=  const=FloorDistance  OutDataTypeStr=boolean
  Constant : Constant  Value=true
  Constant{1..2,7,10,17} (5 alike) : Constant  Value=0
  Constant18 : Constant  Value=true
  Constant19 : Constant
  Constant20 : Constant  Value=All_Paths
  Constant3 : Constant  Value=false  OutDataTypeStr=boolean
  Constant6 : Constant  Value=All_Num_Poses
  NOT1 : Logic  Operator=NOT  AllPortsSameDT=off  OutDataTypeStr=boolean
  Selector : Selector  NumberOfDimensions=3  InputPortWidth=3  IndexOptions=Select all,Select all,Index vector (port)  Indices=[1 3],1,1  OutputSizes=1,1,1
  Selector1 : Selector  IndexOptions=Index vector (port)  Indices=[1 3]  OutputSizes=1
  Subsystem Reference : Subsystem  ReferencedSubsystem=State_Interpreter
  Terminator : Terminator
  Terminator1 : Terminator
  Terminator2 : Terminator
  Gyro_Angle_Adjustment : Outport
  Steering_Abs_Cmd : Outport  Port=2
  Steering_Rel_Cmd : Outport  Port=3
  Translation_Angle : Outport  Port=4
  Translation_Speed : Outport  Port=5
  Is_Absolute_Translation : Outport  Port=6
  Is_Absolute_Steering : Outport  Port=7
  Spline_Enable : Outport  Port=8
  Spline_Ref_Poses : Outport  Port=9
  Spline_Num_Poses : Outport  Port=10
  Test_Mode : Outport  Port=11
  State_Request_Intake_Shooter : Outport  Port=12
  State_Request_Arm : Outport  Port=13
  Climber_Cmd_Direction : Outport  Port=14
  wires:
  Constant6/1 -> Selector1/1
  Subsystem Reference/5 -> Compare To Zero1/1  "Is_Absolute_Translation"
  Constant2/1 -> Steering_Rel_Cmd/1  "Steering_Rel_Cmd"
  Constant10/1 -> Steering_Abs_Cmd/1  "Steering_Abs_Cmd"
  Constant1/1 -> Gyro_Angle_Adjustment/1  "Gyro_Angle_Adjustment"
  Selector/1 -> Spline_Ref_Poses/1  "Spline_Ref_Poses"
  Selector1/1 -> Spline_Num_Poses/1  "Spline_Num_Poses"
  Chassis_Y/1 -> Terminator/1
  Chassis_X/1 -> Terminator1/1
  Constant7/1 -> Translation_Angle/1  "Translation_Angle"
  Subsystem Reference/6 -> Translation_Speed/1  "Translation_Speed"
  Subsystem Reference/3 -> Selector/2, Selector1/2  "Spline_ID"
  NOT1/1 -> Is_Absolute_Steering/1  "Is_Absolute_Steering"
  Constant3/1 -> Test_Mode/1  "Test_Mode"
  Subsystem Reference/4 -> State_Request_Arm/1  "State_Request_Arm"
  Subsystem Reference/1 -> State_Request_Intake_Shooter/1  "State_Request_Intake_Shooter"
  CompareToFloor/1 -> Terminator2/1  "Line_Sensor_Boolean"
  Line_Sensor_TOF_Range/1 -> CompareToFloor/1
  Constant17/1 -> Climber_Cmd_Direction/1  "Climber_Cmd_Direction"
  Auto_ID/1 -> Subsystem Reference/7
  Constant/1 -> Subsystem Reference/6
  PriorityList/1 -> Subsystem Reference/1
  Constant18/1 -> Subsystem Reference/5
  Constant19/1 -> Subsystem Reference/3
  Robot_Reached_Destination/1 -> NOT1/1, Subsystem Reference/2
  IsWaitingForCommand/1 -> Subsystem Reference/4
  Constant20/1 -> Selector/1
  Subsystem Reference/2 -> Compare To Zero/1  "Spline_Enable"
  Compare To Zero/1 -> Spline_Enable/1  "Spline_Enable"
  Compare To Zero1/1 -> Is_Absolute_Translation/1  "Is_Absolute_Translation"

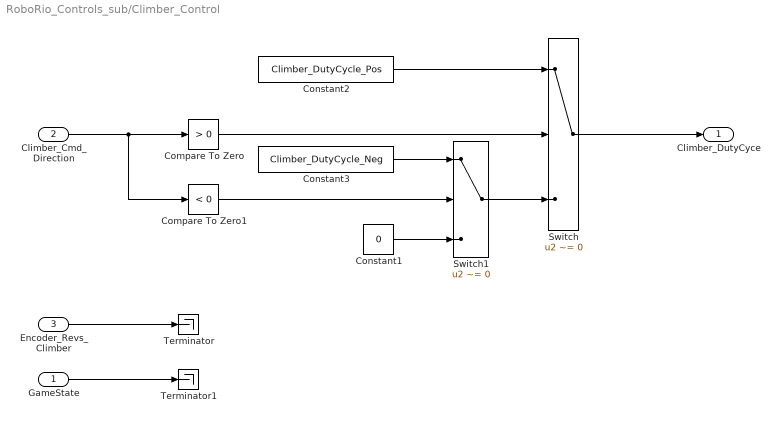
== system RoboRio_Controls_sub/Climber_Control ==
  GameState : Inport
  Climber_Cmd_Direction : Inport  Port=2
  Encoder_Revs_Climber : Inport  Port=3
  Compare To Zero : simulink/Logic and Bit Operations/Compare To Zero  relop=>  OutDataTypeStr=boolean
  Compare To Zero1 : simulink/Logic and Bit Operations/Compare To Zero  relop=<  OutDataTypeStr=boolean
  Constant1 : Constant  Value=0
  Constant2 : Constant  Value=Climber_DutyCycle_Pos
  Constant3 : Constant  Value=Climber_DutyCycle_Neg
  Switch : Switch  Criteria=u2 ~= 0  SaturateOnIntegerOverflow=off  InputSameDT=off
  Switch1 : Switch  Criteria=u2 ~= 0  SaturateOnIntegerOverflow=off  InputSameDT=off
  Terminator : Terminator
  Terminator1 : Terminator
  Climber_DutyCyce : Outport
  wires:
  GameState/1 -> Terminator1/1
  Encoder_Revs_Climber/1 -> Terminator/1
  Switch/1 -> Climber_DutyCyce/1
  Constant3/1 -> Switch1/1
  Constant2/1 -> Switch/1
  Constant1/1 -> Switch1/3
  Compare To Zero1/1 -> Switch1/2
  Compare To Zero/1 -> Switch/2
  Climber_Cmd_Direction/1 -> Compare To Zero/1, Compare To Zero1/1
  Switch1/1 -> Switch/3

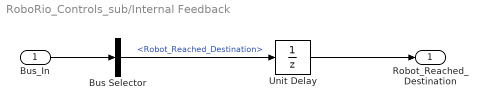
== system RoboRio_Controls_sub/Internal Feedback ==
  Bus_In : Inport
  Bus Selector : BusSelector  OutputSignals=Robot_Reached_Destination
  Unit Delay : UnitDelay  SampleTime=-1  HasFrameUpgradeWarning=on
  Robot_Reached_Destination : Outport
  wires:
  Unit Delay/1 -> Robot_Reached_Destination/1
  Bus Selector/1 -> Unit Delay/1  "<Robot_Reached_Destination>"
  Bus_In/1 -> Bus Selector/1
